simulink model "PVESsystem"  (R2024a)
settings: Solver=FixedStepDiscrete  StartTime=0.0  StopTime=5  FixedStep=1e-6  MaxStep=1e-6  RelTol=1e-3
libraries: spsSeriesRLCBranchLib x7, spsMultimeterLib x4, spsPVArrayLib x2, SignalEditorBlockLib x2, spsDiodeLib x1, spsMosfetLib x1, spsCurrentMeasurementLib x1, eePwmGenerator x1, spsVoltageMeasurementLib x1, sps_lib x1
settings Model: Creator=admin  LastModifiedBy=ZE
settings SolverCC: AllowMultiTaskInputOutput=on
settings ModelReferenceCC: EnableParallelModelReferenceBuilds=on
settings SFSimCC: SimTargetLang=C++  GPUAcceleration=on  SimDLTargetLibrary=cudnn

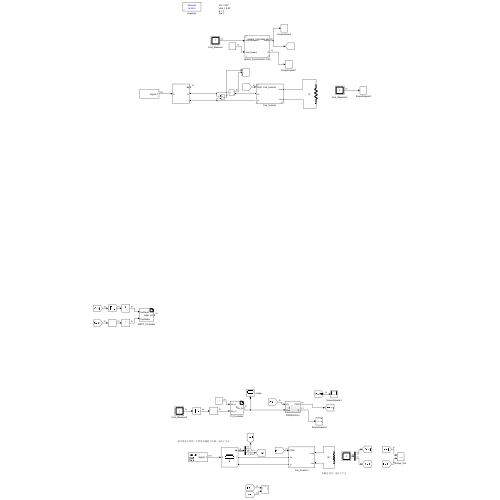
[thumbnail: Simulink's stored preview of the top-level diagram]
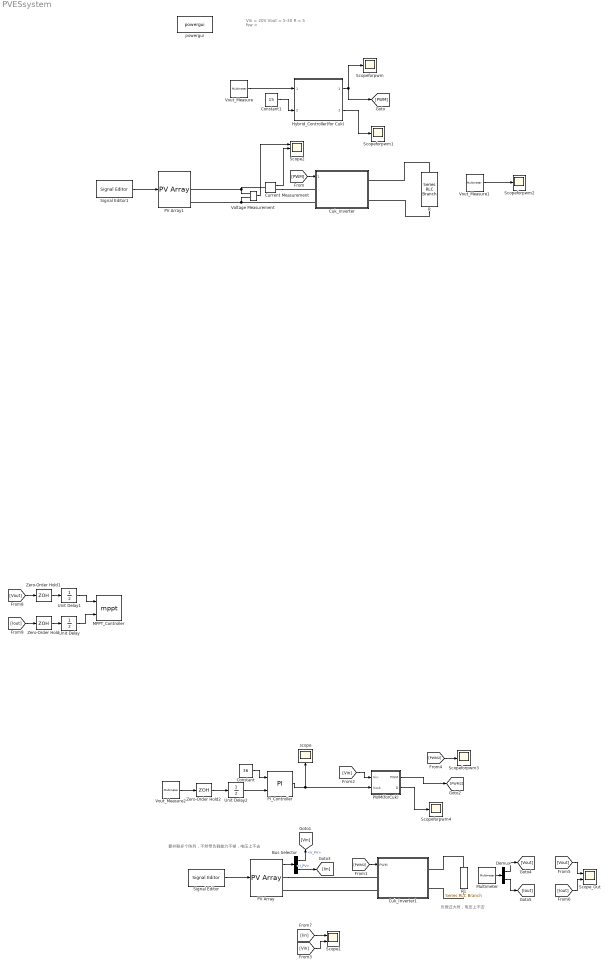
== system PVESsystem ==
  note: 要并联多个阵列，不然带负载能力不够，电压上不去
  note: Vin = 20V
      | Vout = 5-30
      | R = 5
      | fsw =
  note: 负载过大时，电压上不去
  Bus Selector : BusSelector  OutputSignals=V_PV,I_PV
  Constant : Constant  Value=36
  Constant1 : Constant  Value=15
  Cuk_Inverter : Subsystem  ReferencedSubsystem=Cuk_Inverter  Vin=30  Vout_Expect=40  Fsw=100e3  detaIL1=0.1  detaIL2=0.1  detaUC1=0.1  detaUC2=0.1
  Cuk_Inverter1 : Subsystem  mask{Vin=30, Vout_Expect=40, Fsw=100e3, detaIL1=0.1, detaIL2=0.1, detaUC1=0.1, detaUC2=0.1}
      mask prompts: Fsw "Switch Frequency"; detaIL1 "电感纹波"; detaIL2 "电感纹波"; detaUC1 "电压纹波"; detaUC2 "电压纹波"
      mask DialogControl ParameterGroupVar Prompt: 参数
  Current Measurement : spsCurrentMeasurementLib/Current Measurement  PhasorSimulation=off  OutputType=Complex  PSBequivalent=0
  Demux : Demux  Outputs=2
  Hybrid_Controller(for Cuk) : Subsystem  ReferencedSubsystem=Hybrid_Controller_for_Cuk  Vout_Expect=20  Vin=30  Fsw=100e3
  MPPT_Controller : S-Function  FunctionName=mppt  SFunctionModules=mppt_wrapper.cpp  SFunctionDeploymentMode=off  EnableBusSupport=off  mask(S-Function Builder){}
      mask help: Simulink:masks:SFunctionBuilder_MD
      mask init:
      | val = [[.9  0.75 0.75 1 1 .9 .9 1]',[1 1 0.75 0.75 .9 .9 1 .9]'];try , sys = get_param(gcb,'SfunBuilderFcnName');if isempty(sys), sys = get_param(gcb,'FunctionName'); end,catch, sys = get_param(gcb,'FunctionName'); end
      settings: CopyFcn=set_param(gcbh,'LinkStatus','none')  OpenFcn=sfunctionwizard(gcbh)
      mask Display:
      | plot(val(:,1),val(:,2))
      | disp(sys)
      | port_label('input',1,sprintf('%s', 'IpvRead'),'interpreter','tex')
      | port_label('input',2,sprintf('%s', 'VpvRead'),'interpreter','tex')
      | port_label('output',1,sprintf('%s', 'y0'),'interpreter','tex')
  Multimeter : spsMultimeterLib/Multimeter  L=4  sel=[2 4]  yselected={}  Gain=[1 1]  OutputType=Complex  PlotAtSimulationStop=off  PhasorSimulation=off
  PI_Controller : S-Function  FunctionName=PI  SFunctionModules=PI_wrapper.cpp  SFunctionDeploymentMode=off  EnableBusSupport=off  mask(S-Function Builder){}
      mask help: Simulink:masks:SFunctionBuilder_MD
      mask init: same as PVESsystem/MPPT_Controller
      settings: CopyFcn=set_param(gcbh,'LinkStatus','none')  OpenFcn=sfunctionwizard(gcbh)
      mask Display:
      | plot(val(:,1),val(:,2))
      | disp(sys)
      | port_label('input',1,sprintf('%s', 'Vo\_e'),'interpreter','tex')
      | port_label('input',2,sprintf('%s', 'Vo\_m'),'interpreter','tex')
      | port_label('output',1,sprintf('%s', 'Vo\_pi'),'interpreter','tex')
  PV Array : spsPVArrayLib/PV Array  Npar=10  Nser=1  PlotType=array @ 1000 W/m2 & specified temperatures  S_vec="[ 1000  500  100 ]"  Temp_C_vec="[ 45 25  ]"  ModuleName=A10Green Technology A10J-S72-175  PlotWhenSelected=off  Pm=175.0914  Ncell=72  Voc=43.99  Isc=5.17  Vm=36.63  Im=4.78  beta_Voc_pc=-0.3616  alpha_Isc_pc=0.041509  beta_Voc=-0.15907  alpha_Isc=0.002146  IL=5.178  I0=1.7842e-10  nI=0.98852  Rsh=249.6758  Rs=0.38412  RobustModel=on  RobustCellTemperature=25  BAL=on  Tc=1e-6  Tfilter=5e-5
  PV Array1 : spsPVArrayLib/PV Array  Npar=5  Nser=2  PlotType=array @ 1000 W/m2 & specified temperatures  S_vec="[ 1000  500  100 ]"  Temp_C_vec="[ 45 25  ]"  ModuleName=A10Green Technology A10J-S72-175  PlotWhenSelected=off  Pm=175.0914  Ncell=72  Voc=43.99  Isc=5.17  Vm=36.63  Im=4.78  beta_Voc_pc=-0.3616  alpha_Isc_pc=0.041509  beta_Voc=-0.15907  alpha_Isc=0.002146  IL=5.178  I0=1.7842e-10  nI=0.98852  Rsh=249.6758  Rs=0.38412  RobustModel=on  RobustCellTemperature=25  BAL=on  Tc=1e-6  Tfilter=5e-5
  PWM(forCuk) : Subsystem
  R : spsSeriesRLCBranchLib/Series RLC Branch  LConnTagsString=__new0  RConnTagsString=__new0  BranchType=R  Resistance=5  Inductance=1e-3  SetiL0=off  InitialCurrent=0  Capacitance=1e-6  Setx0=off  InitialVoltage=0  Measurements=Branch voltage and current
  R1 : spsSeriesRLCBranchLib/Series RLC Branch  LConnTagsString=__new0  RConnTagsString=__new0  BranchType=R  Resistance=20  Inductance=1e-3  SetiL0=off  InitialCurrent=0  Capacitance=1e-6  Setx0=off  InitialVoltage=0  Measurements=Branch voltage and current
  Scope1 : Scope  NumInputPorts=2
  Scope2 : Scope  NumInputPorts=3
  Scope_Out : Scope  NumInputPorts=2
  Scopeforpwm{,1..4} (5 alike) : Scope
  Signal Editor : SignalEditorBlockLib/Signal Editor  FileName=C:\Users\ZE\Desktop\simulink_workspace\PV_ES_System\solar_Ir.mat  ActiveScenario=Scenario  ActiveSignal=Signal 1  IsBus=off  OutputBusObjectStr=Bus: BusObject  SampleTime=0  OutputAfterFinalValue=Holding final value  Unit=inherit  PreserveSignalName=on  ApplySigPropsToAllScenarios=on  ApplySigPropsToAllSignals=off
  Signal Editor1 : SignalEditorBlockLib/Signal Editor  FileName=C:\Users\ZE\Desktop\simulink_workspace\PV_ES_System\solar_Ir.mat  ActiveScenario=Scenario  ActiveSignal=Signal 1  IsBus=off  OutputBusObjectStr=Bus: BusObject  SampleTime=0  OutputAfterFinalValue=Holding final value  Unit=inherit  PreserveSignalName=on  ApplySigPropsToAllScenarios=on  ApplySigPropsToAllSignals=off
  Unit Delay : UnitDelay  SampleTime=-1  HasFrameUpgradeWarning=on
  Unit Delay1 : UnitDelay  SampleTime=-1  HasFrameUpgradeWarning=on
  Unit Delay2 : UnitDelay  SampleTime=-1  HasFrameUpgradeWarning=on
  Voltage Measurement : spsVoltageMeasurementLib/Voltage Measurement  PhasorSimulation=off  OutputType=Complex  PSBequivalent=0
  Vout_Measure : spsMultimeterLib/Multimeter  L=4  sel=1  yselected={}  Gain=1  OutputType=Complex  PlotAtSimulationStop=off  PhasorSimulation=off
  Vout_Measure1 : spsMultimeterLib/Multimeter  L=4  sel=[1 3]  yselected={}  Gain=[1 1]  OutputType=Complex  PlotAtSimulationStop=off  PhasorSimulation=off
  Vout_Measure2 : spsMultimeterLib/Multimeter  L=4  sel=2  yselected={}  Gain=1  OutputType=Complex  PlotAtSimulationStop=off  PhasorSimulation=off
  Zero-Order Hold : ZeroOrderHold  SampleTime=-1
  Zero-Order Hold1 : ZeroOrderHold  SampleTime=-1
  Zero-Order Hold2 : ZeroOrderHold  SampleTime=-1
  powergui : sps_lib/powergui  Priority=1  SimulationMode=Discrete  SampleTime=1e-6  frequency=60  Iterations=50  frequencyindice=0  Pbase=100e6  ErrMax=1e-4  UnitsV=kV  UnitsW=MW  buscounter=0  FunctionMessages=off  echomessages=off  EnableUseOfTLC=off  CurrentSourceSwitches=off  DisableSnubberDevices=off  DisableRonSwitches=off  DisableVfSwitches=off  DisplayEquations=off  AutomaticDiscreteSolvers=off  SolverType=Tustin/Backward Euler (TBE)  Interpol=off  ExternalGateDelay=off  methode=off  Ts=100  x0status=blocks  SPID=on  SwTol=0  HookPort=off  NonlinearTolerance=1e-4  nMaxIteration=100  ContinueOnMaxIteration=off  RestoreLinks=warning  ResistiveCurrentMeasurement=off  Frange=[0:2:500]  Ylog=off  Xlog=on  ShowGrid=off  save=off  variable=ZData  structure=0  ZoomFFT=off  StartTime=0.0  cycles=1  DisplayStyle=1  fundamental=60  FreqAxis=off  MaxFrequency=1000  frequencyindicesteady=1  RmsSteady=1  display=off
  scope : Scope
  wires:
  Vout_Measure/1 -> Hybrid_Controller(for Cuk)/1
  Hybrid_Controller(for Cuk)/1 -> Scopeforpwm/1, [PWM]
  [PWM] -> Cuk_Inverter/1
  Voltage Measurement/1 -> Scope2/1
  Current Measurement/1 -> Scope2/2
  Constant1/1 -> Hybrid_Controller(for Cuk)/2
  [PWM2] -> Cuk_Inverter1/1(PWM)
  Signal Editor/1 -> PV Array/1
  PWM(forCuk)/1(PWM) -> [PWM2]
  [PWM2] -> Scopeforpwm3/1
  PV Array/1 -> Bus Selector/1
  Bus Selector/1 -> [Vin]  "<V_PV>"
  Bus Selector/2 -> [Iin]  "<I_PV>"
  Multimeter/1 -> Demux/1
  [Iin] -> Scope1/1
  [Vin] -> Scope1/2
  [Vout] -> Zero-Order Hold1/1
  Zero-Order Hold1/1 -> Unit Delay1/1
  [Iout] -> Zero-Order Hold/1
  Zero-Order Hold/1 -> Unit Delay/1
  Unit Delay1/1 -> MPPT_Controller/1
  Unit Delay/1 -> MPPT_Controller/2
  Demux/1 -> [Vout]
  Demux/2 -> [Iout]
  [Vout] -> Scope_Out/1
  [Iout] -> Scope_Out/2
  PI_Controller/1 -> scope/1, PWM(forCuk)/2(Vout)
  Constant/1 -> PI_Controller/1
  Signal Editor1/1 -> PV Array1/1
  Hybrid_Controller(for Cuk)/2 -> Scopeforpwm1/1
  Vout_Measure1/1 -> Scopeforpwm2/1
  Vout_Measure2/1 -> Zero-Order Hold2/1
  PWM(forCuk)/2(D) -> Scopeforpwm4/1
  [Vin] -> PWM(forCuk)/1(Vin)
  Zero-Order Hold2/1 -> Unit Delay2/1
  Unit Delay2/1 -> PI_Controller/2
  connections:
  R/LConn1 -- Cuk_Inverter/RConn1
  R/RConn1 -- Cuk_Inverter/RConn2
  Current Measurement/LConn1 -- Voltage Measurement/LConn1 -- PV Array1/RConn1
  Voltage Measurement/LConn2 -- PV Array1/RConn2 -- Cuk_Inverter/LConn2
  Current Measurement/RConn1 -- Cuk_Inverter/LConn1
  R1/LConn1 -- Cuk_Inverter1/RConn1
  R1/RConn1 -- Cuk_Inverter1/RConn2
  PV Array/RConn1 -- Cuk_Inverter1/LConn1
  Cuk_Inverter1/LConn2 -- PV Array/RConn2

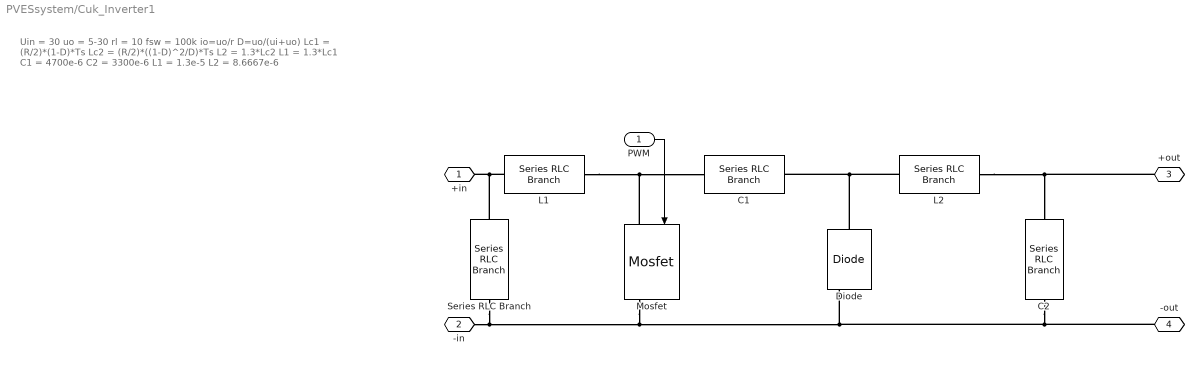
== system PVESsystem/Cuk_Inverter1 ==
  note: Uin = 30
      | uo = 5-30
      | rl = 10
      | fsw = 100k
      | io=uo/r
      |
      | D=uo/(ui+uo)
      | Lc1 = (R/2)*(1-D)*Ts
      | Lc2 = (R/2)*((1-D)^2/D)*Ts
      | L2 = 1.3*Lc2
      | L1 = 1.3*Lc1
      | C1 = 4700e-6
      | C2 = 3300e-6
      |
      | L1 = 1.3e-5
      | L2 = 8.6667e-6
  PWM : Inport
  C1 : spsSeriesRLCBranchLib/Series RLC Branch  LConnTagsString=__new0  RConnTagsString=__new0  BranchType=C  Resistance=1  Inductance=1e-3  SetiL0=off  InitialCurrent=0  Capacitance=0.0047  Setx0=off  InitialVoltage=0  Measurements=None
  C2 : spsSeriesRLCBranchLib/Series RLC Branch  LConnTagsString=__new0  RConnTagsString=__new0  BranchType=C  Resistance=1  Inductance=1e-3  SetiL0=off  InitialCurrent=0  Capacitance=0.01  Setx0=off  InitialVoltage=0  Measurements=None
  Diode : spsDiodeLib/Diode  Ron=0.001  Lon=0  Vf=0.8  IC=0  UseSnubber=0  Rs=500  Cs=250e-9  Measurements=on
  L1 : spsSeriesRLCBranchLib/Series RLC Branch  LConnTagsString=__new0  RConnTagsString=__new0  BranchType=L  Resistance=1  Inductance=1e-3  SetiL0=off  InitialCurrent=0  Capacitance=1e-6  Setx0=off  InitialVoltage=0  Measurements=None
  L2 : spsSeriesRLCBranchLib/Series RLC Branch  LConnTagsString=__new0  RConnTagsString=__new0  BranchType=L  Resistance=1  Inductance=8.6667e-6  SetiL0=off  InitialCurrent=0  Capacitance=1e-6  Setx0=off  InitialVoltage=0  Measurements=None
  Mosfet : spsMosfetLib/Mosfet  Ron=0.1  Lon=0  Rd=0.01  Vfd=0  IC=0  Rs=1e5  Cs=inf  Measurements=on
  Series RLC Branch : spsSeriesRLCBranchLib/Series RLC Branch  LConnTagsString=__new0  RConnTagsString=__new0  BranchType=C  Resistance=1  Inductance=1e-3  SetiL0=off  InitialCurrent=0  Capacitance=1e-5  Setx0=off  InitialVoltage=0  Measurements=None
  +in : PMIOPort  Side=Left
  -in : PMIOPort  Port=2  Side=Left
  +out : PMIOPort  Port=3  Side=Right
  -out : PMIOPort  Port=4  Side=Right
  wires:
  PWM/1 -> Mosfet/1
  connections:
  L2/RConn1 -- +out/RConn1 -- C2/LConn1
  L2/LConn1 -- Diode/LConn1 -- C1/RConn1
  L1/LConn1 -- Series RLC Branch/LConn1 -- +in/RConn1
  L1/RConn1 -- Mosfet/LConn1 -- C1/LConn1
  Mosfet/RConn1 -- -in/RConn1 -- Series RLC Branch/RConn1 -- -out/RConn1 -- C2/RConn1 -- Diode/RConn1

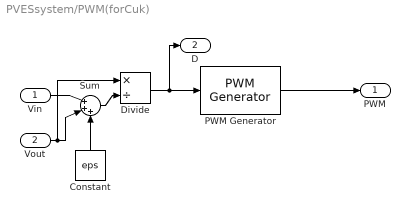
== system PVESsystem/PWM(forCuk) ==
  Vin : Inport
  Vout : Inport  Port=2
  Constant : Constant  Value=eps
  Divide : Product  Inputs=*/
  PWM Generator : eePwmGenerator/PWM Generator  CarrCount=Up  Tper=1e-5  Tdelay=0  Ts=1e-6
  Sum : Sum  Inputs=|+++
  PWM : Outport
  D : Outport  Port=2
  wires:
  PWM Generator/1 -> PWM/1
  Vin/1 -> Sum/1
  Vout/1 -> Divide/1, Sum/2
  Sum/1 -> Divide/2
  Constant/1 -> Sum/3
  Divide/1 -> D/1, PWM Generator/1
